simulink model "matlabinduction1"  (R2022b)
settings: Solver=ode45  StartTime=0.0  StopTime=1  RelTol=1e-3
libraries: spsIGBTDiodeLib x6, spsRMSLib x2, spsAsynchronousMachineSIUnitsLib x1, spsDCVoltageSourceLib x1, simulink x1, spsThreePhaseVIMeasurementLib x1, spspowerguiLib x1
settings Model: Creator=Nagagopika  LastModifiedBy=durai
settings OptimizationCC: ReuseModelBlockBuffer=on

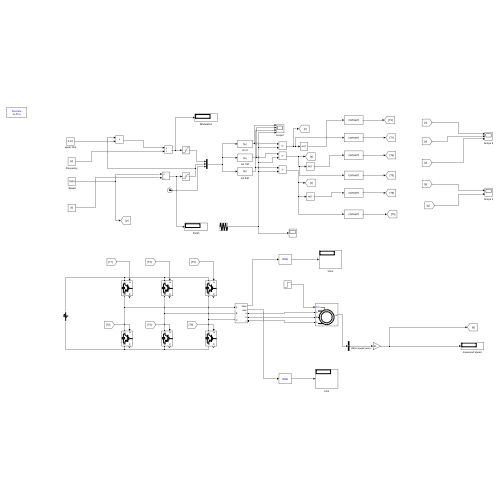
[thumbnail: Simulink's stored preview of the top-level diagram]
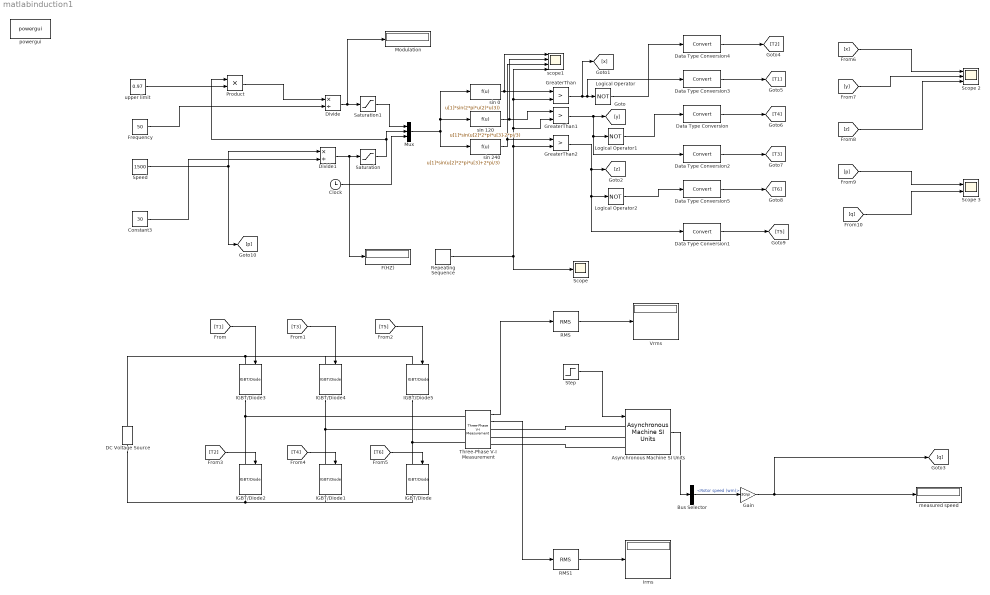
== system matlabinduction1 ==
  " Speed" : Constant  Value=1500
  Asynchronous Machine SI Units : spsAsynchronousMachineSIUnitsLib/Asynchronous Machine SI Units  RotorType=Squirrel-cage  PresetModel=No  MechanicalLoad=Torque Tm  ShowDetailedParameters=on  ReferenceFrame=Rotor  Units=SI  MeasurementBus=off  NominalParameters=[1.845e+04 400 50]  VoltageRatio=1  Stator=[0.5968 0.0003495]  Rotor=[0.6258 0.005473]  Cage1=[0.4155 0.002066]  Cage2=[0.4168 0.0003495]  Lm=0.0354  Mechanical=[0.05 0.005879 2]  PolePairs=2  InitialConditions=[0 0 0 0 0 0 0 0]  SimulateSaturation=off  Saturation=[14.03593122, 27.81365428, 53.79336849, 72.68890987, 97.98006896, 148.6815601, 215.7428561, 302.9841135, 428.7778367 ; 230, 322, 414, 460, 506, 552, 598, 644, 690]  LoadFlowParameters=1492000  TsPowergui=0  TsBlock=-1  IterativeModel=Trapezoidal non iterative  IterativeDiscreteModel=Trapezoidal non iterative  Pmec=1.492e+006
  Bus Selector : BusSelector  OutputSignals=Mechanical.Rotor speed (wm)
  Clock : Clock
  Constant3 : Constant  Value=30
  DC Voltage Source : spsDCVoltageSourceLib/DC Voltage Source  Amplitude=600  Measurements=None
  Data Type Conversion{,1..5} (6 alike) : DataTypeConversion  SaturateOnIntegerOverflow=off  RndMeth=Floor
  Divide : Product  Inputs=*/
  Divide1 : Product  Inputs=*/
  F(HZ) : Display
  Frequency : Constant  Value=50
  Gain : Gain  Gain=30/pi
  GreaterThan : RelationalOperator  Operator=>  OutDataTypeStr=boolean  RndMeth=Simplest  InputSameDT=off
  GreaterThan1 : RelationalOperator  Operator=>  OutDataTypeStr=boolean  RndMeth=Simplest  InputSameDT=off
  GreaterThan2 : RelationalOperator  Operator=>  OutDataTypeStr=boolean  RndMeth=Simplest  InputSameDT=off
  IGBT/Diode{,1..5} (6 alike) : spsIGBTDiodeLib/IGBT//Diode  Ron=1e-3  Rs=1e5  Cs=inf  Measurements=on
  Irms : Display
  Logical Operator : Logic  Operator=NOT  AllPortsSameDT=off  OutDataTypeStr=boolean
  Logical Operator1 : Logic  Operator=NOT  AllPortsSameDT=off  OutDataTypeStr=boolean
  Logical Operator2 : Logic  Operator=NOT  AllPortsSameDT=off  OutDataTypeStr=boolean
  Modulation : Display
  Mux : Mux  Inputs=3
  Product : Product
  RMS : spsRMSLib/RMS  TrueRMS=on  Freq=50  RMSInit=120  Ts=0
  RMS1 : spsRMSLib/RMS  TrueRMS=on  Freq=50  RMSInit=120  Ts=0
  Repeating Sequence : simulink/Sources/Repeating Sequence  rep_seq_t="[0 1/(4*1050)  1/(2*1050)  3/(4*1050)  1/1050]"  rep_seq_y=[0 1 0 -1 0]
  Saturation : Saturate  UpperLimit=75  LowerLimit=0
  Saturation1 : Saturate  UpperLimit=0.97  LowerLimit=0.3
  Scope : Scope
  Scope 2 : Scope  NumInputPorts=3
  Scope 3 : Scope  NumInputPorts=2
  Step : Step  Time=5  Before=10  After=15  SampleTime=0
  Three-Phase V-I Measurement : spsThreePhaseVIMeasurementLib/Three-Phase V-I Measurement  VoltageMeasurement=phase-to-phase  SetLabelV=off  LabelV=Vabc  Vpu=off  VpuLL=off  CurrentMeasurement=yes  SetLabelI=off  LabelI=Iabc  Ipu=off  Pbase=100e6  Vbase=500e3  OutputType=Complex  PhasorSimulation=off  PSBequivalent=0
  Vrms : Display
  measured speed : Display
  powergui : spspowerguiLib/powergui  Priority=1  SimulationMode=Discrete  SampleTime=10e-6  frequency=60  Iterations=50  frequencyindice=50  Pbase=100e6  ErrMax=1e-4  UnitsV=kV  UnitsW=MW  buscounter=0  FunctionMessages=off  echomessages=off  EnableUseOfTLC=off  CurrentSourceSwitches=off  DisableSnubberDevices=off  DisableRonSwitches=off  DisableVfSwitches=off  DisplayEquations=off  AutomaticDiscreteSolvers=off  SolverType=Tustin/Backward Euler (TBE)  Interpol=off  ExternalGateDelay=off  methode=off  Ts=100  x0status=blocks  SPID=on  SwTol=0  HookPort=off  NonlinearTolerance=1e-4  nMaxIteration=100  ContinueOnMaxIteration=off  RestoreLinks=warning  ResistiveCurrentMeasurement=off  Frange=[0:2:500]  Ylog=off  Xlog=on  ShowGrid=off  save=off  variable=ZData  structure=0  ZoomFFT=off  StartTime=0.0  cycles=1  DisplayStyle=1  fundamental=60  FreqAxis=off  MaxFrequency=1000  frequencyindicesteady=1  RmsSteady=1  display=off
  scope1 : Scope  NumInputPorts=4
  sin 0 : Fcn  Expr=u[1]*sin(2*pi*u(2)*u(3))
  sin 120 : Fcn  Expr=u[1]*sin(u[2]*2*pi*u[3]-2*pi/3)
  sin 240 : Fcn  Expr=u[1]*sin(u[2]*2*pi*u[3]+2*pi/3)
  upper limit : Constant  Value=0.97
  wires:
  [T1] -> IGBT/Diode3/1
  [T3] -> IGBT/Diode4/1
  [T5] -> IGBT/Diode5/1
  [T2] -> IGBT/Diode2/1
  [T4] -> IGBT/Diode1/1
  [T6] -> IGBT/Diode/1
  [x] -> Scope 2/1
  [y] -> Scope 2/2
  [z] -> Scope 2/3
  [p] -> Scope 3/1
  [q] -> Scope 3/2
  Step/1 -> Asynchronous Machine SI Units/1
  GreaterThan/1 -> [x], Data Type Conversion3/1, Logical Operator/1
  GreaterThan1/1 -> Data Type Conversion2/1, Logical Operator1/1, [y]
  GreaterThan2/1 -> [z], Data Type Conversion1/1, Logical Operator2/1
  Bus Selector/1 -> Gain/1  "<Rotor speed (wm)>"
  Gain/1 -> [q], measured speed/1
  RMS1/1 -> Irms/1
  Divide/1 -> Modulation/1, Saturation1/1
  Divide1/1 -> F(HZ)/1, Saturation/1
  upper limit/1 -> Product/2
  Product/1 -> Divide/1
  Frequency/1 -> Divide/2
  " Speed"/1 -> Divide1/1, [p]
  Constant3/1 -> Divide1/2
  Saturation1/1 -> Mux/1
  Saturation/1 -> Product/1, Mux/2
  Clock/1 -> Mux/3
  sin 0/1 -> scope1/1, GreaterThan/1
  sin 240/1 -> scope1/3, GreaterThan2/1
  Mux/1 -> sin 240/1, sin 120/1, sin 0/1
  Repeating Sequence/1 -> GreaterThan1/2, GreaterThan/2, scope1/4, GreaterThan2/2, Scope/1
  sin 120/1 -> scope1/2, GreaterThan1/1
  Logical Operator/1 -> Data Type Conversion4/1
  Logical Operator1/1 -> Data Type Conversion/1
  Logical Operator2/1 -> Data Type Conversion5/1
  Data Type Conversion4/1 -> [T2]
  Data Type Conversion3/1 -> [T1]
  Data Type Conversion/1 -> [T4]
  Data Type Conversion2/1 -> [T3]
  Data Type Conversion5/1 -> [T6]
  Data Type Conversion1/1 -> [T5]
  Three-Phase V-I Measurement/1 -> RMS/1
  Three-Phase V-I Measurement/2 -> RMS1/1
  RMS/1 -> Vrms/1
  Asynchronous Machine SI Units/1 -> Bus Selector/1
  connections:
  DC Voltage Source/RConn1 -- IGBT/Diode3/LConn1 -- IGBT/Diode4/LConn1 -- IGBT/Diode5/LConn1
  Three-Phase V-I Measurement/LConn1 -- IGBT/Diode2/LConn1 -- IGBT/Diode3/RConn1
  Three-Phase V-I Measurement/LConn2 -- IGBT/Diode1/LConn1 -- IGBT/Diode4/RConn1
  Three-Phase V-I Measurement/LConn3 -- IGBT/Diode/LConn1 -- IGBT/Diode5/RConn1
  DC Voltage Source/LConn1 -- IGBT/Diode2/RConn1 -- IGBT/Diode/RConn1 -- IGBT/Diode1/RConn1
  Asynchronous Machine SI Units/LConn1 -- Three-Phase V-I Measurement/RConn1
  Asynchronous Machine SI Units/LConn2 -- Three-Phase V-I Measurement/RConn2
  Asynchronous Machine SI Units/LConn3 -- Three-Phase V-I Measurement/RConn3
